simulink model "AL_model_YAW"  (R2023b)
settings: Solver=FixedStepAuto  StartTime=0.0  StopTime=t(end)  FixedStep=0.002  RelTol=1e-3
settings Model: Creator=franc  LastModifiedBy=franc

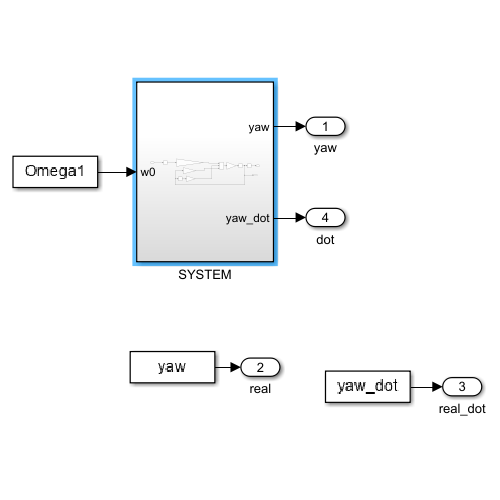
[thumbnail: Simulink's stored preview of the top-level diagram]
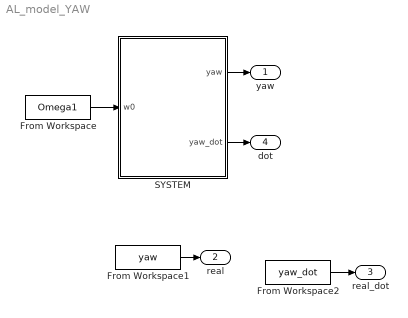
== system AL_model_YAW ==
  From Workspace : FromWorkspace  VariableName=Omega1
  From Workspace1 : FromWorkspace  VariableName=yaw
  From Workspace2 : FromWorkspace  VariableName=yaw_dot
  SYSTEM : Subsystem
  yaw : Outport
  real : Outport  Port=2
  real_dot : Outport  Port=3
  dot : Outport  Port=4
  wires:
  From Workspace/1 -> SYSTEM/1(w0)
  SYSTEM/1(yaw) -> yaw/1
  From Workspace1/1 -> real/1
  From Workspace2/1 -> real_dot/1
  SYSTEM/2(yaw_dot) -> dot/1

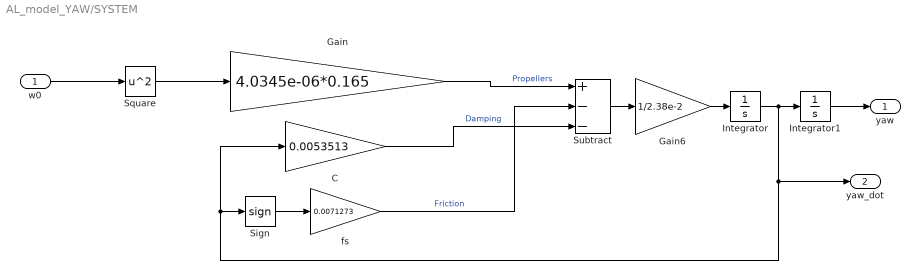
== system AL_model_YAW/SYSTEM ==
  w0 : Inport
  C : Gain  Gain=0.0053513
  Gain : Gain  Gain=4.0345e-06*0.165
  Gain6 : Gain  Gain=1/2.38e-2
  Integrator : Integrator
  Integrator1 : Integrator
  Sign : Signum
  Square : Math  Operator=square
  Subtract : Sum  Inputs=+--
  fs : Gain  Gain=0.0071273
  yaw : Outport
  yaw_dot : Outport  Port=2
  wires:
  Gain6/1 -> Integrator/1
  Gain/1 -> Subtract/1  "Propellers"
  Integrator1/1 -> yaw/1
  Integrator/1 -> Integrator1/1, yaw_dot/1, C/1, Sign/1
  Subtract/1 -> Gain6/1
  C/1 -> Subtract/3  "Damping"
  Sign/1 -> fs/1
  Square/1 -> Gain/1
  fs/1 -> Subtract/2  "Friction"
  w0/1 -> Square/1
